simulink model "model"  (Simulink 7.4)
settings: Solver=ode45  StartTime=0  StopTime=50  MaxStep=2e-2  RelTol=1e-3
values from neighbouring files (symbols this model uses):
  Bm = 3e-6    (= 3e-06)    [beammodelparameters.m]
  g = 9.8    [beammodelparameters.m]
  Gv = 2    [beammodelparameters.m]
  Jeff = Jm + Jg + Js    (= 5.66e-05)    [beammodelparameters.m]
  K = (2/5)*(R/r)^2    (= 1.11111111111)    [beammodelparameters.m]
  Ks = 10    [beammodelparameters.m]
  Kt = 0.125    [beammodelparameters.m]
  Lm = 7.5e-3    (= 0.0075)    [beammodelparameters.m]
  M = 1 + (2/5)*(R/r)^2    (= 2.11111111111)    [beammodelparameters.m]
  N = 100    [beammodelparameters.m]
  Rm = 4    [beammodelparameters.m]
  theta_o = 0.1    [beammodelparameters.m]
  Vlim = 50    [beammodelparameters.m]
  x_o = 0.25    [beammodelparameters.m]
undefined symbols (not defined in the file or in its folder): Cd, ck, Cn
libraries: simulink x1
settings Model: Creator=Duane  LastModifiedBy=Cam  ExtModeAutoUpdateStatusClock=off
settings DebuggingCC: SolverPrmCheckMsg=none

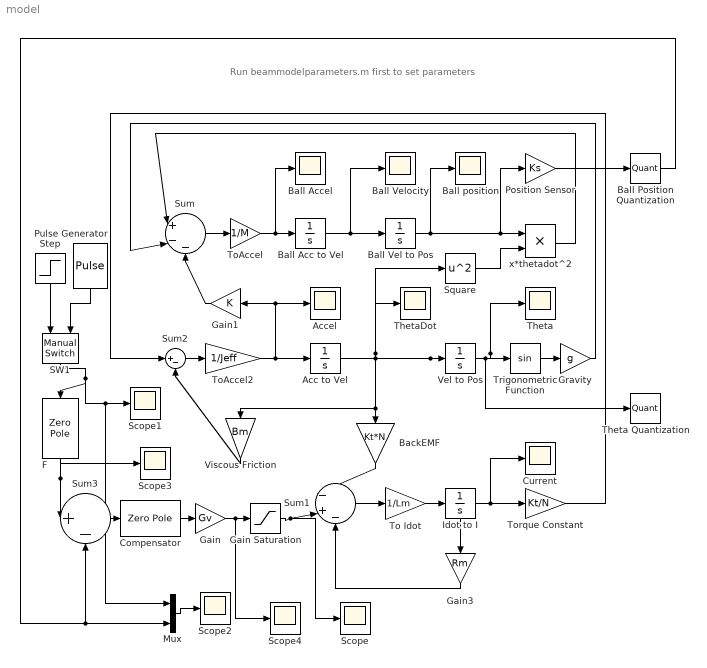
== system model ==
  note: Run beammodelparameters.m first to set parameters
  Acc to Vel : Integrator
  Accel : Scope
      settings: SaveName=ScopeData5
  BackEMF : Gain  Gain=Kt*N  ParameterDataType=fixdt(1, 16)  ParameterScaling=2^0  OutDataType=fixdt(1, 16)  OutScaling=2^0
  Ball Acc to Vel : Integrator
  Ball Accel : Scope
      settings: SaveName=ScopeData6
  Ball Position Quantization : Quantizer  QuantizationInterval=Xquant
  Ball Vel to Pos : Integrator  InitialCondition=x_o
  Ball Velocity : Scope
  Ball position : Scope
  Compensator : ZeroPole  Zeros=Cn  Poles=Cd  Gain=ck
  Current : Scope
      settings: SaveName=ScopeData4
  F : ZeroPole  Zeros=[]  Poles=[-1 -1]
  Gain : Gain  Gain=Gv  ParameterDataType=fixdt(1, 16)  ParameterScaling=2^0  OutDataType=fixdt(1, 16)  OutScaling=2^0
  Gain Saturation : Saturate  UpperLimit=Vlim  LowerLimit=-Vlim  OutDataType=fixdt(1, 16)  OutScaling=2^0
  Gain1 : Gain  Gain=K  ParameterDataType=fixdt(1, 16)  ParameterScaling=2^0  OutDataType=fixdt(1, 16)  OutScaling=2^0
  Gain3 : Gain  Gain=Rm  ParameterDataType=fixdt(1, 16)  ParameterScaling=2^0  OutDataType=fixdt(1, 16)  OutScaling=2^0
  Gravity : Gain  Gain=g  ParameterDataType=fixdt(1, 16)  ParameterScaling=2^0  OutDataType=fixdt(1, 16)  OutScaling=2^0
  Idot to I : Integrator
  Mux : Mux  Inputs=2
  Position Sensor : Gain  Gain=Ks  ParameterDataType=fixdt(1, 16)  ParameterScaling=2^0  OutDataType=fixdt(1, 16)  OutScaling=2^0
  Pulse Generator : DiscretePulseGenerator  PulseType=Time based  Amplitude=1  Period=8  PulseWidth=50  PhaseDelay=0  SampleTime=1
  SW1 : simulink/Signal Routing/Manual Switch  SystemSampleTime=-1  sw=1  action=0  varsize=off
  Scope{,1..4} (5 alike) : Scope
      Scope settings: SaveName=ScopeData7
      Scope1 settings: SaveName=ScopeData8
      Scope2 settings: SaveName=ScopeData9
      Scope3 settings: SaveName=ScopeData10
      Scope4 settings: SaveName=ScopeData11
  Square : Math  Operator=square  OutDataType=fixdt(1, 16)  OutScaling=2^0  SaturateOnIntegerOverflow=on
  Step : Step  After=-2.5  SampleTime=0
  Sum : Sum  Inputs=|+--  OutDataType=fixdt(1, 16)  OutScaling=2^0
  Sum1 : Sum  Inputs=|-+-  OutDataType=fixdt(1, 16)  OutScaling=2^0
  Sum2 : Sum  Inputs=|+-  OutDataType=fixdt(1, 16)  OutScaling=2^0
  Sum3 : Sum  Inputs=|+-  OutDataType=fixdt(1, 16)  OutScaling=2^0
  Theta : Scope
      settings: SaveName=ScopeData2
  Theta Quantization : Quantizer  QuantizationInterval=Tquant
  ThetaDot : Scope
      settings: SaveName=ScopeData3
  To Idot : Gain  Gain=1/Lm  ParameterDataType=fixdt(1, 16)  ParameterScaling=2^0  OutDataType=fixdt(1, 16)  OutScaling=2^0
  ToAccel : Gain  Gain=1/M  ParameterDataType=fixdt(1, 16)  ParameterScaling=2^0  OutDataType=fixdt(1, 16)  OutScaling=2^0
  ToAccel2 : Gain  Gain=1/Jeff  ParameterDataType=fixdt(1, 16)  ParameterScaling=2^0  OutDataType=fixdt(1, 16)  OutScaling=2^0
  Torque Constant : Gain  Gain=Kt/N  ParameterDataType=fixdt(1, 16)  ParameterScaling=2^0  OutDataType=fixdt(1, 16)  OutScaling=2^0
  Trigonometric Function : Trigonometry
  Vel to Pos : Integrator  InitialCondition=theta_o
  Viscous Friction : Gain  Gain=Bm  ParameterDataType=fixdt(1, 16)  ParameterScaling=2^0  OutDataType=fixdt(1, 16)  OutScaling=2^0
  x*thetadot^2 : Product  Inputs=**  OutDataType=fixdt(1, 16)  OutScaling=2^-10
  wires:
  Ball Acc to Vel/1 -> Ball Vel to Pos/1, Ball Velocity/1
  Vel to Pos/1 -> Theta/1, Trigonometric Function/1, Theta Quantization/1
  ToAccel/1 -> Ball Acc to Vel/1, Ball Accel/1
  Sum/1 -> ToAccel/1
  Square/1 -> x*thetadot^2/2
  Ball Vel to Pos/1 -> Ball position/1, x*thetadot^2/1, Position Sensor/1
  x*thetadot^2/1 -> Sum/1
  Acc to Vel/1 -> Vel to Pos/1, Square/1, Viscous Friction/1, BackEMF/1, ThetaDot/1
  Gain3/1 -> Sum1/3
  Idot to I/1 -> Torque Constant/1, Gain3/1, Current/1
  To Idot/1 -> Idot to I/1
  Sum1/1 -> To Idot/1
  Trigonometric Function/1 -> Gravity/1
  Gravity/1 -> Sum/2
  Gain Saturation/1 -> Sum1/2, Scope/1
  ToAccel2/1 -> Acc to Vel/1, Accel/1, Gain1/1
  Sum2/1 -> ToAccel2/1
  Viscous Friction/1 -> Sum2/2
  Position Sensor/1 -> Ball Position Quantization/1
  Torque Constant/1 -> Sum2/1
  Gain1/1 -> Sum/3
  BackEMF/1 -> Sum1/1
  Compensator/1 -> Gain/1
  Sum3/1 -> Compensator/1
  Ball Position Quantization/1 -> Mux/2, Sum3/2
  Gain/1 -> Gain Saturation/1, Scope4/1
  Mux/1 -> Scope2/1
  Step/1 -> SW1/1
  Pulse Generator/1 -> SW1/2
  SW1/1 -> Mux/1, Scope1/1, F/1
  F/1 -> Sum3/1, Scope3/1
